simulink model "lookup_nD_TestGen9"  (R2017b)
settings: Solver=FixedStepDiscrete  StartTime=0.0  StopTime=10.0  RelTol=1e-3
model workspace (MAT data in the model file):
  LUTObjLKnD9 = Simulink.LookupTable
  LUTObjLKnD9.Table = Simulink.lookuptable.Table
  LUTObjLKnD9.Table.Value = [10.2006563775  99.1225713804  102.073086964  62.9444094206  78.1964371724; 103.969060195  123.203847871  18.9526484012  19.7825950445  77.0655386285; 20.4268484765  47.7732964452  111.879509264  86.415536164  97.9267084978]
  LUTObjLKnD9.Table.Dimensions = [3 5]
  LUTObjLKnD9.Table.DataType = 'double'
  LUTObjLKnD9.Table.FieldName = 'Table'
  LUTObjLKnD9.Breakpoints(1) = Simulink.lookuptable.Breakpoint
  LUTObjLKnD9.Breakpoints(1).Value = [34.7213483504; 57.5775185354; 123.844382949]
  LUTObjLKnD9.Breakpoints(1).TunableSizeName = 'N1'
  LUTObjLKnD9.Breakpoints(1).Dimensions = [3 1]
  LUTObjLKnD9.Breakpoints(1).DataType = 'double'
  LUTObjLKnD9.Breakpoints(1).FieldName = 'BP1'
  LUTObjLKnD9.Breakpoints(2) = Simulink.lookuptable.Breakpoint
  LUTObjLKnD9.Breakpoints(2).Value = [7.33164667661; 30.0141641189; 54.5688692346; 56.2270461747; 63.4017251445]
  LUTObjLKnD9.Breakpoints(2).TunableSizeName = 'N2'
  LUTObjLKnD9.Breakpoints(2).Dimensions = [5 1]
  LUTObjLKnD9.Breakpoints(2).DataType = 'double'
  LUTObjLKnD9.Breakpoints(2).FieldName = 'BP2'
  LUTObjLKnD9.SupportTunableSize = 0
  LUTObjLKnD9.StructTypeInfo = Simulink.lookuptable.StructTypeInfo
  LUTObjLKnD9.StructTypeInfo.Name = 'LUT'
  LUTObjLKnD9.StructTypeInfo.DataScope = 'Auto'
settings Model: Creator=ktrinh  LastModifiedBy=ktrinh
settings DebuggingCC: ParameterOverflowMsg=none

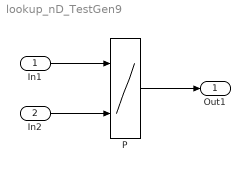
== system lookup_nD_TestGen9 ==
  In1 : Inport  OutMin=0  OutMax=127  PortDimensions=1
  In2 : Inport  Port=2  OutMin=0  OutMax=127
  P : Lookup_n-D  DataSpecification=Lookup table object  LookupTableObject=LUTObjLKnD9  BreakpointsForDimension3=[5, 7]  Table=reshape(repmat([4 5 6;16 19 20;10 18 23],1,2),[3,3,2])  InterpMethod=Nearest  ExtrapMethod=Clip  InternalRulePriority=Speed  OutDataTypeStr=double  SaturateOnIntegerOverflow=on  InputSameDT=on
  Out1 : Outport
  wires:
  In1/1 -> P/1
  In2/1 -> P/2
  P/1 -> Out1/1
